simulink model "ex4"  (R2020a)
settings: Solver=FixedStepAuto  StartTime=0.0  StopTime=10  RelTol=1e-3
libraries: androidsensorlib x9, androiduilib x9
settings Model: Creator=corte  LastModifiedBy=corte
settings DataIOCC: ReturnWorkspaceOutputs=off
settings OptimizationCC: EnhancedBackFolding=on  PassReuseOutputArgsAs=Individual arguments  ZeroExternalMemoryAtStartup=off  ZeroInternalMemoryAtStartup=off  MaxStackSize=64  OptimizeBlockOrder=speed  DifferentSizesBufferReuse=on  OptimizationCustomize=off  EfficientTunableParamExpr=on
settings DebuggingCC: ParameterTunabilityLossMsg=error
settings HardwareCC: ProdBitPerPointer=32  ProdBitPerSizeT=32  ProdBitPerPtrDiffT=32  ProdLargestAtomicInteger=Long  ProdLargestAtomicFloat=Double  ProdWordSize=32  ProdHWDeviceType=ARM Compatible->ARM Cortex
settings SFSimCC: MATLABDynamicMemAlloc=off
settings RTWCC: SystemTargetFile=ert.tlc  HardwareBoard=Android Device  TemplateMakefile=ert_default_tmf  RTWVerbose=off  Toolchain=Android SDK/NDK Tools
settings CodeAppCC: ForceParamTrailComments=on  IgnoreCustomStorageClasses=off  OperatorAnnotations=on  SimulinkDataObjDesc=on  SFDataObjDesc=on  InsertBlockDesc=on
settings ERTTargetCC: SupportContinuousTime=on

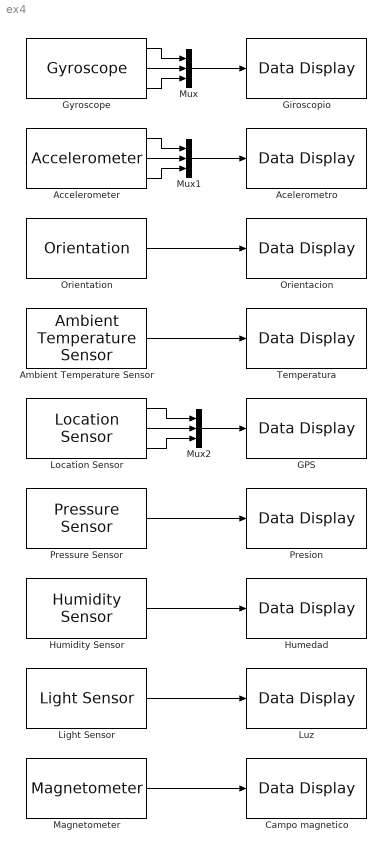
== system ex4 ==
  Accelerometer : androidsensorlib/Accelerometer  OutputVector=off  SampleTime=0.1  BlockPlatform=Android
      settings: SourceProductBaseCode=ANDROID
  Acelerometro : androiduilib/Data Display  DataDisplayId=ex4/Acelerometro  Format=Float  Precision=1  SimulateUsing=Code generation  blockPlatform=Android
      settings: SourceProductBaseCode=ANDROID
  Ambient Temperature Sensor : androidsensorlib/Ambient Temperature Sensor  SampleTime=0.1  BlockPlatform=Android
      settings: SourceProductBaseCode=ANDROID
  Campo magnetico : androiduilib/Data Display  DataDisplayId=ex4/Campo_magnetico  Format=Float  Precision=1  SimulateUsing=Code generation  blockPlatform=Android
      settings: SourceProductBaseCode=ANDROID
  GPS : androiduilib/Data Display  DataDisplayId=ex4/GPS  Format=Float  Precision=1  SimulateUsing=Code generation  blockPlatform=Android
      settings: SourceProductBaseCode=ANDROID
  Giroscopio : androiduilib/Data Display  DataDisplayId=ex4/Giroscopio  Format=Float  Precision=1  SimulateUsing=Code generation  blockPlatform=Android
      settings: SourceProductBaseCode=ANDROID
  Gyroscope : androidsensorlib/Gyroscope  OutputVector=off  SampleTime=0.1  BlockPlatform=Android
      settings: SourceProductBaseCode=ANDROID
  Humedad : androiduilib/Data Display  DataDisplayId=ex4/Humedad  Format=Float  Precision=1  SimulateUsing=Code generation  blockPlatform=Android
      settings: SourceProductBaseCode=ANDROID
  Humidity Sensor : androidsensorlib/Humidity Sensor  SampleTime=0.1  BlockPlatform=Android
      settings: SourceProductBaseCode=ANDROID
  Light Sensor : androidsensorlib/Light Sensor  SampleTime=0.1  BlockPlatform=Android
      settings: SourceProductBaseCode=ANDROID
  Location Sensor : androidsensorlib/Location Sensor  OutputVector=off  SampleTime=0.1  BlockPlatform=Android
      settings: SourceProductBaseCode=ANDROID
  Luz : androiduilib/Data Display  DataDisplayId=ex4/Luz  Format=Float  Precision=1  SimulateUsing=Code generation  blockPlatform=Android
      settings: SourceProductBaseCode=ANDROID
  Magnetometer : androidsensorlib/Magnetometer  SampleTime=0.1  SimulateUsing=Code generation
      settings: SourceProductBaseCode=ANDROID
  Mux : Mux  Inputs=3
  Mux1 : Mux  Inputs=3
  Mux2 : Mux  Inputs=3
  Orientacion : androiduilib/Data Display  DataDisplayId=ex4/Orientacion  Format=Float  Precision=1  SimulateUsing=Code generation  blockPlatform=Android
      settings: SourceProductBaseCode=ANDROID
  Orientation : androidsensorlib/Orientation  SampleTime=0.1  SimulateUsing=Code generation
      settings: SourceProductBaseCode=ANDROID
  Presion : androiduilib/Data Display  DataDisplayId=ex4/Presion  Format=Float  Precision=1  SimulateUsing=Code generation  blockPlatform=Android
      settings: SourceProductBaseCode=ANDROID
  Pressure Sensor : androidsensorlib/Pressure Sensor  SampleTime=0.1  BlockPlatform=Android
      settings: SourceProductBaseCode=ANDROID
  Temperatura : androiduilib/Data Display  DataDisplayId=ex4/Temperatura  Format=Float  Precision=1  SimulateUsing=Code generation  blockPlatform=Android
      settings: SourceProductBaseCode=ANDROID
  wires:
  Mux/1 -> Giroscopio/1
  Gyroscope/2 -> Mux/2
  Gyroscope/1 -> Mux/1
  Gyroscope/3 -> Mux/3
  Accelerometer/3 -> Mux1/3
  Accelerometer/1 -> Mux1/1
  Accelerometer/2 -> Mux1/2
  Mux1/1 -> Acelerometro/1
  Orientation/1 -> Orientacion/1
  Ambient Temperature Sensor/1 -> Temperatura/1
  Mux2/1 -> GPS/1
  Location Sensor/2 -> Mux2/2
  Location Sensor/1 -> Mux2/1
  Location Sensor/3 -> Mux2/3
  Pressure Sensor/1 -> Presion/1
  Humidity Sensor/1 -> Humedad/1
  Light Sensor/1 -> Luz/1
  Magnetometer/1 -> Campo magnetico/1
